simulink model "e5_Quadrotor_stable_nn_cex"  (R2020a)
settings: Solver=FixedStepAuto  StartTime=0.0  StopTime=options.T_train  FixedStep=options.dt  RelTol=1e-6
undefined symbols (not defined in the file or in its folder): options, Quad
libraries: neural x179, simulink x3
(part 7 of 10)

== system e5_Quadrotor_stable_nn_cex/NN_cex_1/Layer 2/Delays 1 ==
  "p{2}" : Inport  PortDimensions=50
      mask Display: e = 0.06;c1 = [120 230 180]/255;c2 = ([120 230 180]+0)/(256+128);c3 = ([120 230 180]+128)/(256+128);patch([0 1 1 0],[0 0 1 1],c1);patch([0 1 1 1-e 1-e 0+e],[0 0 1 1-e 0+e 0+e],c2);patch([0 0 1 1-e 0+e 0+e],[0 1 1 1-e 1-e 0+e],c3);plot([0 1 1 0 0],[0 0 1 1 0]);
  mux : Mux  Inputs=1
      mask Display: e = 0.06;c1 = [120 150 230]/255;c2 = ([120 150 230]+0)/383;c3 = ([120 150 230]+128)/383;patch([0 1 1 0],[0 0 1 1],c1);patch([0 1 1 1-e 1-e 0+e],[0 0 1 1-e 0+e 0+e],c2);patch([0 0 1 1-e 0+e 0+e],[0 1 1 1-e 1-e 0+e],c3);plot([0 1 1 0 0],[0 0 1 1 0]);disp('Mux')
  "pd{2,1}" : Outport
      mask Display: e = 0.06;c1 = [120 230 180]/255;c2 = ([120 230 180]+0)/(256+128);c3 = ([120 230 180]+128)/(256+128);patch([0 1 1 0],[0 0 1 1],c1);patch([0 1 1 1-e 1-e 0+e],[0 0 1 1-e 0+e 0+e],c2);patch([0 0 1 1-e 0+e 0+e],[0 1 1 1-e 1-e 0+e],c3);plot([0 1 1 0 0],[0 0 1 1 0]);
  wires:
  "p{2}"/1 -> mux/1
  mux/1 -> "pd{2,1}"/1

== system e5_Quadrotor_stable_nn_cex/NN_cex_1/Layer 2/LW{2,1} ==
  "ad{2,1}" : Inport  PortDimensions=50
      mask Display: e = 0.06;c1 = [120 230 180]/255;c2 = ([120 230 180]+0)/(256+128);c3 = ([120 230 180]+128)/(256+128);patch([0 1 1 0],[0 0 1 1],c1);patch([0 1 1 1-e 1-e 0+e],[0 0 1 1-e 0+e 0+e],c2);patch([0 0 1 1-e 0+e 0+e],[0 1 1 1-e 1-e 0+e],c3);plot([0 1 1 0 0],[0 0 1 1 0]);
  "IW{2,1}(1,:)'" : Constant  Value=[-0.0088685301363819642184171954113480751402676105499267578125;-0.475176525636941848862448978252359665930271148681640625;-0.06647124940185501762446307338905171491205692291259765625;-0.1239059849711940664018783309074933640658855438232421875;0.032635022619955177114459132781121297739446163177490234375;0.01583916238122483333139456362914643250405788421630859375;-0.27280857013441550673604751864331774413585662841796875;-0.0031640968694437638687733116427125423797406256198883056640625;0.223718246479297722117962621268816292285919189453125;-0.394448205193596468376426855684258043766021728515625;0.0979383343874088707625702454606653191149234771728515625;-0.53425641285417591053175101478700526058673858642578125;-0.03146462718389790580442166856300900690257549285888671875;-0.239740076844939975497794648617855273187160491943359375;-0.440191595975097438309120434496435336768627166748046875;-0.66366872940875432096419217486982233822345733642578125;-0.10444158073413657705774681971888639964163303375244140625;0.55638869101991239585203175010974518954753875732421875;0.331489331826144428827518595426226966083049774169921875;0.60432691051748033128632187072071246802806854248046875;0.1289300914259262353933621625401428900659084320068359375;-0.322220670294381561493679555496782995760440826416015625;-1.2284029185784193227704008677392266690731048583984375;-0.58967119568664927431456135309417732059955596923828125;-0.0060351614102806712403026523361404542811214923858642578125;0.09623664814751171914242178218046319670975208282470703125;0.64319280324351602029508967461879365146160125732421875;0.61766341328172791325101798065588809549808502197265625;-0.847320852952669678614938675309531390666961669921875;-0.625730442492045568769754027016460895538330078125;-0.88157264982928662533367969444952905178070068359375;-0.57075826696425846495941414104891009628772735595703125;-0.77851626064118573111727528157643973827362060546875;0.70362500226065105568551416581613011658191680908203125;0.5450944965061557123675584080046974122524261474609375;1.16584476611400322809686258551664650440216064453125;0.68163889471687733045968116130097769200801849365234375;-0.139178826639824781974397183148539625108242034912109375;0.57538559923232635018308656071894802153110504150390625;-0.84010338979454513008704452659003436565399169921875;1.642364503369627026785337875480763614177703857421875;-0.0881088539475056442551448299127514474093914031982421875;0.0874097000117176892164394530482240952551364898681640625;0.2085951939359249884820002307606046088039875030517578125;0.642820243629548482289237654185853898525238037109375;0.351359414295920824411467719983193092048168182373046875;-0.63290393665018707114455764894955791532993316650390625;-0.7574217553083990583928652995382435619831085205078125;0.95372305881493690815631225632387213408946990966796875;0.10191035180150519179331780605934909544885158538818359375]
      mask Display: e = 0.06;c1 = [120 150 230]/255;c2 = ([120 150 230]+0)/383;c3 = ([120 150 230]+128)/383;patch([0 1 1 0],[0 0 1 1],c1);patch([0 1 1 1-e 1-e 0+e],[0 0 1 1-e 0+e 0+e],c2);patch([0 0 1 1-e 0+e 0+e],[0 1 1 1-e 1-e 0+e],c3);plot([0 1 1 0 0],[0 0 1 1 0]);disp('weights');
  "IW{2,1}(2,:)'" : Constant  Value=[0.092370250412365073611198340586270205676555633544921875;0.09270531154826489039777470679837279021739959716796875;-0.2364786142915533684316642393241636455059051513671875;0.039897396312396526951715713948942720890045166015625;0.240566123944577825444213203809340484440326690673828125;-0.147079610050850018154733334085904061794281005859375;-0.6618189333725206235925497821881435811519622802734375;-0.498375918980829613058602944875019602477550506591796875;0.109700635576793548153773372177965939044952392578125;0.0455589308588773278518857523522456176578998565673828125;-0.93628476908035251913275942570180632174015045166015625;0.279178053284372562625748059872421436011791229248046875;0.1809035697566074019082549284576089121401309967041015625;-0.90884274192985348150841673486866056919097900390625;-0.0114196202164255911082335614992189221084117889404296875;-0.25654036859093298783562886455911211669445037841796875;0.0711678189737881827792165267965174280107021331787109375;-0.548115626917613507629312152857892215251922607421875;-0.04253389232205771752770573357338435016572475433349609375;-0.18090648231674866242002508442965336143970489501953125;-0.484359210653714067351671701544546522200107574462890625;-0.31653598865277732254952525181579403579235076904296875;1.0840943165254282032350374720408581197261810302734375;0.9933511044620362273604996516951359808444976806640625;0.307551335541762560499279288706020452082157135009765625;-0.1741277372226967823376497790377470664680004119873046875;0.09766993107279310637469649236663826741278171539306640625;-0.44364455943896385914371194303384982049465179443359375;-0.101649841012934893935693025923683308064937591552734375;0.03227070195956018017202637793161557056009769439697265625;0.06026669960555774974153564471635036170482635498046875;-0.033846763822895579998384363307195599190890789031982421875;0.62708327655847295734048429949325509369373321533203125;-0.4086407096254289772474521669209934771060943603515625;-0.23618596679244518998785906660486944019794464111328125;-0.573600653695542472831903069163672626018524169921875;-0.33761730603049622256861539426608942449092864990234375;0.36134775893436710259010169465909712016582489013671875;0.5768777693348192681099817491485737264156341552734375;0.6708632328480927942138123398763127624988555908203125;-0.339738918025521086097029410666436888277530670166015625;-0.60007981003736954317417939819279126822948455810546875;0.06718104714142054956216298933213693089783191680908203125;-0.60274288301443468274243286941782571375370025634765625;0.4657142703865775335003718282678164541721343994140625;-1.190348107955280010372689503128640353679656982421875;-0.316656727339016452749120844600838609039783477783203125;0.403234456146223496642022610103595070540904998779296875;-0.04824704399061445492247202082580770365893840789794921875;0.226941019189561055124926269854768179357051849365234375]
      mask Display: e = 0.06;c1 = [120 150 230]/255;c2 = ([120 150 230]+0)/383;c3 = ([120 150 230]+128)/383;patch([0 1 1 0],[0 0 1 1],c1);patch([0 1 1 1-e 1-e 0+e],[0 0 1 1-e 0+e 0+e],c2);patch([0 0 1 1-e 0+e 0+e],[0 1 1 1-e 1-e 0+e],c3);plot([0 1 1 0 0],[0 0 1 1 0]);disp('weights');
  Mux : Mux  Inputs=2
      mask Display: e = 0.06;c1 = [120 150 230]/255;c2 = ([120 150 230]+0)/383;c3 = ([120 150 230]+128)/383;patch([0 1 1 0],[0 0 1 1],c1);patch([0 1 1 1-e 1-e 0+e],[0 0 1 1-e 0+e 0+e],c2);patch([0 0 1 1-e 0+e 0+e],[0 1 1 1-e 1-e 0+e],c3);plot([0 1 1 0 0],[0 0 1 1 0]);disp('Mux');
  dotprod1 : neural/Weight Functions/dotprod
  dotprod2 : neural/Weight Functions/dotprod
  "lz{2,1}" : Outport
      mask Display: e = 0.06;c1 = [120 230 180]/255;c2 = ([120 230 180]+0)/(256+128);c3 = ([120 230 180]+128)/(256+128);patch([0 1 1 0],[0 0 1 1],c1);patch([0 1 1 1-e 1-e 0+e],[0 0 1 1-e 0+e 0+e],c2);patch([0 0 1 1-e 0+e 0+e],[0 1 1 1-e 1-e 0+e],c3);plot([0 1 1 0 0],[0 0 1 1 0]);
  wires:
  "IW{2,1}(1,:)'"/1 -> dotprod1/1
  "ad{2,1}"/1 -> dotprod1/2, dotprod2/2
  dotprod1/1 -> Mux/1
  "IW{2,1}(2,:)'"/1 -> dotprod2/1
  dotprod2/1 -> Mux/2
  Mux/1 -> "lz{2,1}"/1

== system e5_Quadrotor_stable_nn_cex/NN_online/Layer 1/Delays 1 ==
  "p{1}" : Inport  PortDimensions=20
      mask Display: e = 0.06;c1 = [120 230 180]/255;c2 = ([120 230 180]+0)/(256+128);c3 = ([120 230 180]+128)/(256+128);patch([0 1 1 0],[0 0 1 1],c1);patch([0 1 1 1-e 1-e 0+e],[0 0 1 1-e 0+e 0+e],c2);patch([0 0 1 1-e 0+e 0+e],[0 1 1 1-e 1-e 0+e],c3);plot([0 1 1 0 0],[0 0 1 1 0]);
  mux : Mux  Inputs=1
      mask Display: e = 0.06;c1 = [120 150 230]/255;c2 = ([120 150 230]+0)/383;c3 = ([120 150 230]+128)/383;patch([0 1 1 0],[0 0 1 1],c1);patch([0 1 1 1-e 1-e 0+e],[0 0 1 1-e 0+e 0+e],c2);patch([0 0 1 1-e 0+e 0+e],[0 1 1 1-e 1-e 0+e],c3);plot([0 1 1 0 0],[0 0 1 1 0]);disp('Mux')
  "pd{1,1}" : Outport
      mask Display: e = 0.06;c1 = [120 230 180]/255;c2 = ([120 230 180]+0)/(256+128);c3 = ([120 230 180]+128)/(256+128);patch([0 1 1 0],[0 0 1 1],c1);patch([0 1 1 1-e 1-e 0+e],[0 0 1 1-e 0+e 0+e],c2);patch([0 0 1 1-e 0+e 0+e],[0 1 1 1-e 1-e 0+e],c3);plot([0 1 1 0 0],[0 0 1 1 0]);
  wires:
  "p{1}"/1 -> mux/1
  mux/1 -> "pd{1,1}"/1
